simulink model "Hibrido"  (R2013a)
settings: Solver=FixedStepDiscrete  StartTime=0.0  StopTime=10.0  RelTol=1e-3
settings Model: Creator=Élio  LastModifiedBy=Élio
settings OptimizationCC: InlineParams=on

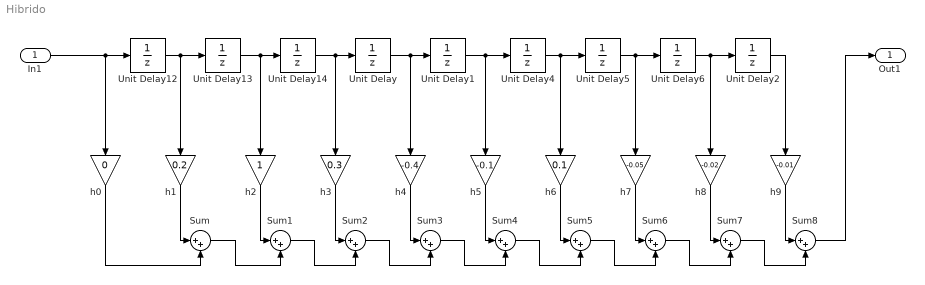
== system Hibrido ==
  In1 : Inport
  Sum{,1..8} (9 alike) : Sum  Inputs=|++
  Unit Delay{,1..2,4..6,12..14} (9 alike) : UnitDelay  SampleTime=-1
  h0 : Gain  Gain=0
  h1 : Gain  Gain=0.2
  h2 : Gain
  h3 : Gain  Gain=0.3
  h4 : Gain  Gain=-0.4
  h5 : Gain  Gain=-0.1
  h6 : Gain  Gain=0.1
  h7 : Gain  Gain=-0.05
  h8 : Gain  Gain=-0.02
  h9 : Gain  Gain=-0.01
  Out1 : Outport
  wires:
  Unit Delay12/1 -> Unit Delay13/1, h1/1
  Unit Delay13/1 -> Unit Delay14/1, h2/1
  Unit Delay14/1 -> Unit Delay/1, h3/1
  Unit Delay/1 -> Unit Delay1/1, h4/1
  Unit Delay1/1 -> Unit Delay4/1, h5/1
  Unit Delay4/1 -> Unit Delay5/1, h6/1
  Unit Delay5/1 -> Unit Delay6/1, h7/1
  Unit Delay6/1 -> Unit Delay2/1, h8/1
  Unit Delay2/1 -> h9/1
  h1/1 -> Sum/1
  h0/1 -> Sum/2
  In1/1 -> Unit Delay12/1, h0/1
  Sum/1 -> Sum1/2
  h2/1 -> Sum1/1
  h3/1 -> Sum2/1
  h4/1 -> Sum3/1
  h5/1 -> Sum4/1
  h6/1 -> Sum5/1
  h7/1 -> Sum6/1
  h8/1 -> Sum7/1
  h9/1 -> Sum8/1
  Sum1/1 -> Sum2/2
  Sum2/1 -> Sum3/2
  Sum3/1 -> Sum4/2
  Sum4/1 -> Sum5/2
  Sum5/1 -> Sum6/2
  Sum6/1 -> Sum7/2
  Sum7/1 -> Sum8/2
  Sum8/1 -> Out1/1
